simulink model "statefdbk_w_observer"  (R2021b)
settings: Solver=VariableStepAuto  StartTime=0.0  StopTime=10  RelTol=1e-3
values from neighbouring files (symbols this model uses):
  C = diag([1,1,1,1,1])    [inv_pendulum.m]
  D = [0 0 0 0 0]'    [inv_pendulum.m]
  K = lqr(A, B, Qr, Rr)    [inv_pendulum.m]
  L = lqe(A, G, C, Qe, Re)    [inv_pendulum.m]
  x0 = [0.1 0 0 0 0]'    [inv_pendulum.m]
undefined symbols (not defined in the file or in its folder): A, B
settings Model: Creator=freed  LastModifiedBy=freed

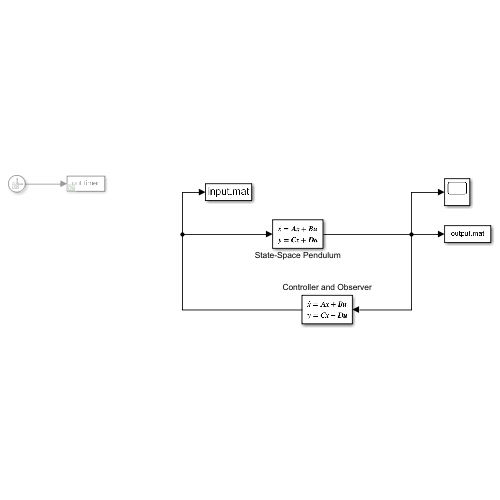
[thumbnail: Simulink's stored preview of the top-level diagram]
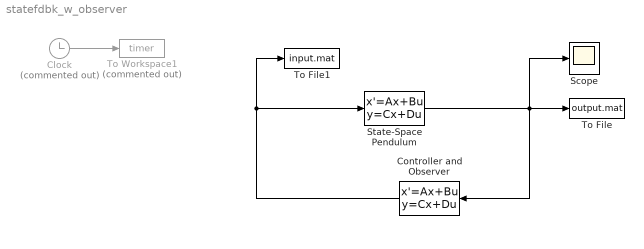
== system statefdbk_w_observer ==
  Clock : Clock  Commented=on
  Controller and Observer : StateSpace  A=A - B*K - L*C  B=L  C=-K  D=[0 0]  InitialCondition=0  ParameterTunability=Unconstrained
  Scope : Scope
  State-Space Pendulum : StateSpace  A=A  B=B  C=C  D=D  InitialCondition=x0  ParameterTunability=Unconstrained
  To File : ToFile  Filename=output.mat  MatrixName=y
  To File1 : ToFile  Filename=input.mat  MatrixName=u
  To Workspace1 : ToWorkspace  Commented=on  VariableName=timer  SaveFormat=Timeseries  SampleTime=-1
  wires:
  Clock/1 -> To Workspace1/1
  State-Space Pendulum/1 -> To File/1, Controller and Observer/1, Scope/1
  Controller and Observer/1 -> To File1/1, State-Space Pendulum/1
